simulink model "fir_filter"  (R2024a)
settings: Solver=VariableStepAuto  StartTime=0.0  StopTime=10.0  RelTol=1e-3
values from neighbouring files (symbols this model uses):
  b = fir1(numtaps-1, fc/(fs/2), 'low', hamming(numtaps))    [param_for_fir_fft.m]
settings Model: Creator=MaxV  LastModifiedBy=MaxV

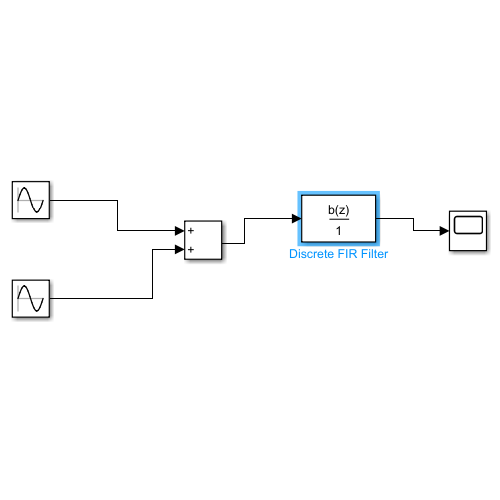
[thumbnail: Simulink's stored preview of the top-level diagram]
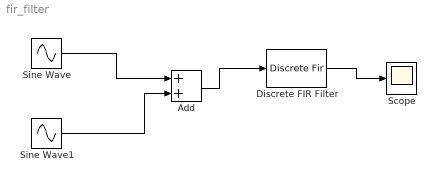
== system fir_filter ==
  Add : Sum
  Discrete FIR Filter : DiscreteFir  Coefficients=b
  Scope : Scope
  Sine Wave : Sin  Amplitude=0.5  Phase=2*pi*120  SampleTime=0
  Sine Wave1 : Sin  Frequency=2*pi*50  SampleTime=0
  wires:
  Sine Wave/1 -> Add/1
  Sine Wave1/1 -> Add/2
  Add/1 -> Discrete FIR Filter/1
  Discrete FIR Filter/1 -> Scope/1
